simulink subsystem "CheckDtnParam"  (R2023b)
settings: Solver=VariableStepAuto  StartTime=0.0  StopTime=10.0  RelTol=1e-3
libraries: simulink x1
settings Model: Creator=dfurodet  LastModifiedBy=dfurodet

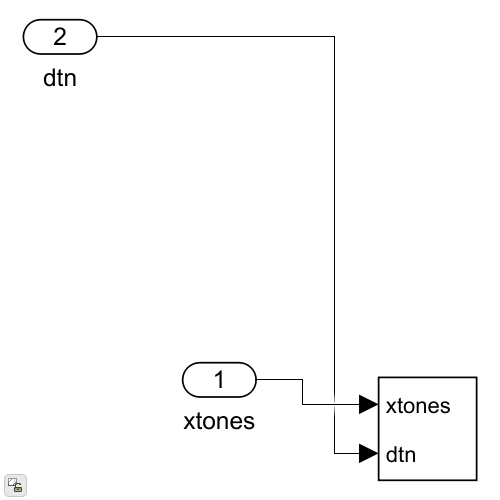
[thumbnail: Simulink's stored preview of the top-level diagram]
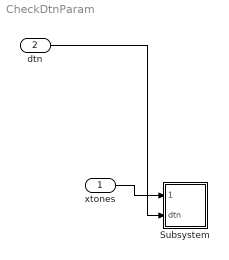
== system CheckDtnParam ==
  xtones : Inport
  dtn : Inport  Port=2
  Subsystem : Subsystem
  wires:
  dtn/1 -> Subsystem/2(dtn)
  xtones/1 -> Subsystem/1(xtones)

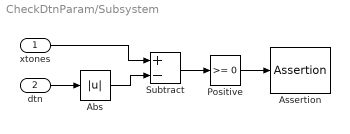
== system CheckDtnParam/Subsystem ==
  xtones : Inport
  dtn : Inport  Port=2
  Abs : Abs  SaturateOnIntegerOverflow=off
  Assertion : Assertion
  Positive : simulink/Logic and Bit Operations/Compare To Zero  relop=>=  OutDataTypeStr=boolean
  Subtract : Sum  Inputs=+-
  wires:
  Subtract/1 -> Positive/1
  Positive/1 -> Assertion/1
  Abs/1 -> Subtract/2
  xtones/1 -> Subtract/1
  dtn/1 -> Abs/1
